simulink subsystem "estimate_RLS_MPC_Model"  (R2024b)
settings: Solver=VariableStepAuto  StartTime=0.0  StopTime=10.0  RelTol=1e-3
undefined symbols (not defined in the file): BallAndPlate_1aixs_tf_d, EKF_u_num, EKF_x_num, EKF_y_num
libraries: slident x4
settings Model: Creator=tshintai  LastModifiedBy=tshintai
settings OptimizationCC: ReuseModelBlockBuffer=off
settings ModelReferenceCC: EnableRefExpFcnMdlSchedulingChecks=on
settings RTWCC: GPUComputeCapability=3.5

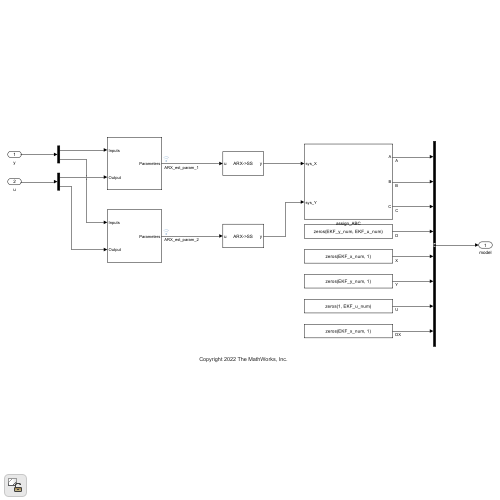
[thumbnail: Simulink's stored preview of the top-level diagram]
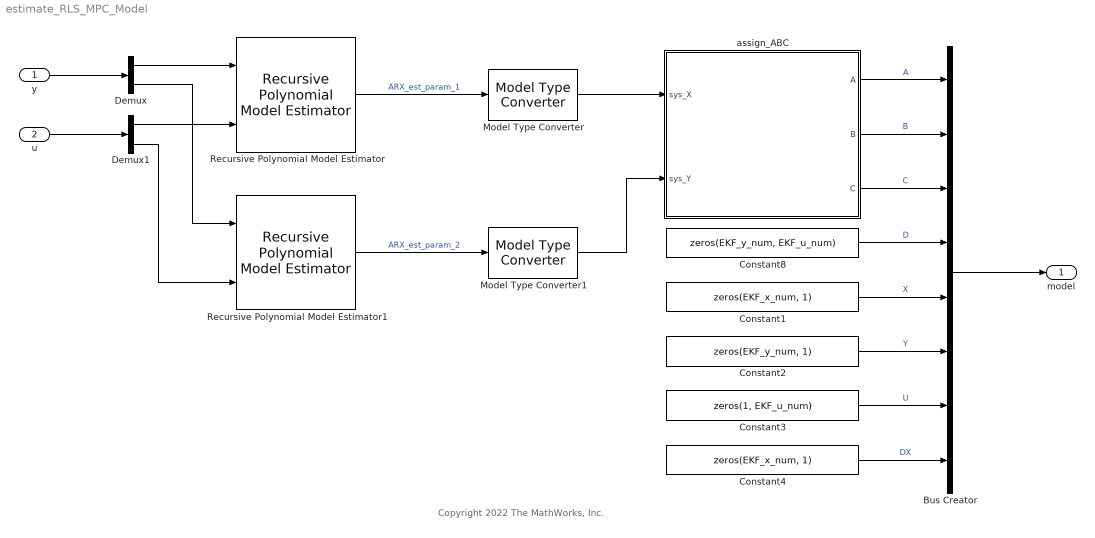
== system estimate_RLS_MPC_Model ==
  note: Copyright 2022 The MathWorks, Inc.
  y : Inport
  u : Inport  Port=2
  Bus Creator : BusCreator  Inputs=8
  Constant1 : Constant  Value=zeros(EKF_x_num, 1)  VectorParams1D=off  OutDataTypeStr=single
  Constant2 : Constant  Value=zeros(EKF_y_num, 1)  VectorParams1D=off  OutDataTypeStr=single
  Constant3 : Constant  Value=zeros(1, EKF_u_num)  VectorParams1D=off  OutDataTypeStr=single
  Constant4 : Constant  Value=zeros(EKF_x_num, 1)  VectorParams1D=off  OutDataTypeStr=single
  Constant8 : Constant  Value=zeros(EKF_y_num, EKF_u_num)  VectorParams1D=off  OutDataTypeStr=single
  Demux : Demux  Outputs=2
  Demux1 : Demux  Outputs=2
  Model Type Converter : slident/Estimators/Model Type Converter  InputModelType=ARX
  Model Type Converter1 : slident/Estimators/Model Type Converter  InputModelType=ARX
  Recursive Polynomial Model Estimator : slident/Estimators/Recursive Polynomial Model Estimator  ModelStructure=ARX  InitialEstimateSource=Internal  A0=BallAndPlate_1aixs_tf_d.Denominator{1}  B0=BallAndPlate_1aixs_tf_d.Numerator{1}  C0=1  D0=1  F0=1  nk=[0 0]  P0=1e-6  InitialInputs=0  InitialOutputs=0  History=Infinite  WindowLength=200  EstimationMethod=Gradient  AdaptationParameter=RLS_adaptive_gain  HasTimeVaryingAdaptationParameter=off  NormalizationBias=eps  OutputError=off  OutputP=off  AddEnablePort=off  InputProcessing=Sample-based  Ts=-1
  Recursive Polynomial Model Estimator1 : slident/Estimators/Recursive Polynomial Model Estimator  ModelStructure=ARX  InitialEstimateSource=Internal  A0=BallAndPlate_1aixs_tf_d.Denominator{1}  B0=BallAndPlate_1aixs_tf_d.Numerator{1}  C0=1  D0=1  F0=1  nk=[0 0]  P0=1e-6  InitialInputs=0  InitialOutputs=0  History=Infinite  WindowLength=200  EstimationMethod=Gradient  AdaptationParameter=RLS_adaptive_gain  HasTimeVaryingAdaptationParameter=off  NormalizationBias=eps  OutputError=off  OutputP=off  AddEnablePort=off  InputProcessing=Sample-based  Ts=-1
  assign_ABC : Subsystem
  model : Outport
  wires:
  Constant2/1 -> Bus Creator/6  "Y"
  assign_ABC/1(A) -> Bus Creator/1  "A"
  assign_ABC/2(B) -> Bus Creator/2  "B"
  assign_ABC/3(C) -> Bus Creator/3  "C"
  Constant8/1 -> Bus Creator/4  "D"
  Constant3/1 -> Bus Creator/7  "U"
  Constant4/1 -> Bus Creator/8  "DX"
  Constant1/1 -> Bus Creator/5  "X"
  Demux/1 -> Recursive Polynomial Model Estimator/1
  Demux1/1 -> Recursive Polynomial Model Estimator/2
  Demux/2 -> Recursive Polynomial Model Estimator1/1
  Demux1/2 -> Recursive Polynomial Model Estimator1/2
  Model Type Converter/1 -> assign_ABC/1(sys_X)
  Model Type Converter1/1 -> assign_ABC/2(sys_Y)
  y/1 -> Demux/1
  u/1 -> Demux1/1
  Recursive Polynomial Model Estimator/1 -> Model Type Converter/1  "ARX_est_param_1"
  Recursive Polynomial Model Estimator1/1 -> Model Type Converter1/1  "ARX_est_param_2"
  Bus Creator/1 -> model/1

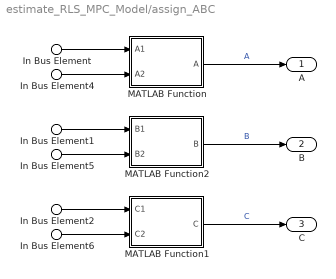
== system estimate_RLS_MPC_Model/assign_ABC ==
  In Bus Element : Inport  PortName=sys_X  Element=A
  In Bus Element1 : Inport  PortName=sys_X  Element=B
  In Bus Element2 : Inport  PortName=sys_X  Element=C
  In Bus Element4 : Inport  Port=2  PortName=sys_Y  Element=A
  In Bus Element5 : Inport  Port=2  PortName=sys_Y  Element=B
  In Bus Element6 : Inport  Port=2  PortName=sys_Y  Element=C
  MATLAB Function : MATLAB Function  TreatAsAtomicUnit=on
  MATLAB Function1 : MATLAB Function  TreatAsAtomicUnit=on
  MATLAB Function2 : MATLAB Function  TreatAsAtomicUnit=on
  A : Outport
  B : Outport  Port=2
  C : Outport  Port=3
  wires:
  MATLAB Function2/1(B) -> B/1  "B"
  In Bus Element1/1 -> MATLAB Function2/1(B1)
  In Bus Element2/1 -> MATLAB Function1/1(C1)
  In Bus Element4/1 -> MATLAB Function/2(A2)
  In Bus Element6/1 -> MATLAB Function1/2(C2)
  In Bus Element5/1 -> MATLAB Function2/2(B2)
  In Bus Element/1 -> MATLAB Function/1(A1)
  MATLAB Function/1(A) -> A/1  "A"
  MATLAB Function1/1(C) -> C/1  "C"

== matlab function estimate_RLS_MPC_Model/assign_ABC/MATLAB Function1 ==
  data: C1 input; C output; C2 input
function C = fcn(C1, C2)
n = size(C1,2);
C = [C1 zeros(1,n);zeros(1,n) C2];

== matlab function estimate_RLS_MPC_Model/assign_ABC/MATLAB Function2 ==
  data: B1 input; B output; B2 input
function B = fcn(B1, B2)
n = size(B1);
B = [B1 zeros(n);zeros(n) B2];

== matlab function estimate_RLS_MPC_Model/assign_ABC/MATLAB Function ==
  data: A1 input; A output; A2 input
function A = fcn(A1, A2)
n = size(A1);
A = [A1 zeros(n);zeros(n) A2];
